simulink model "Mod5Counter"  (R2020a)
settings: Solver=VariableStepAuto  StartTime=0.0  StopTime=10.0  RelTol=1e-3
settings Model: Creator=Admin  LastModifiedBy=Admin

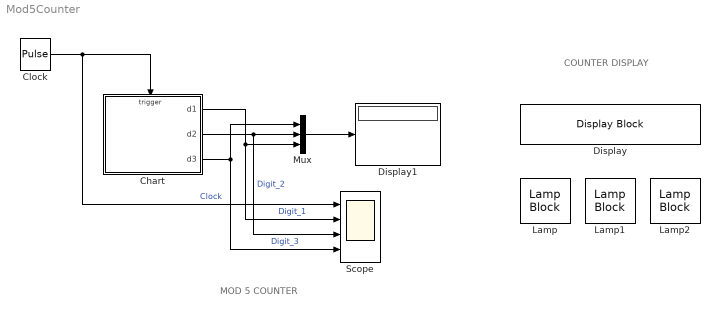
== system Mod5Counter ==
  note: MOD 5 COUNTER
  note: COUNTER DISPLAY
  Chart : Stateflow chart  TreatAsAtomicUnit=on
  Clock : DiscretePulseGenerator  PulseType=Time based  Period=0.5  PulseWidth=50
  Display : DisplayBlock  LabelPosition=Hide  Format=short  Transparency=1
  Display1 : Display
  Lamp : LampBlock
  Lamp1 : LampBlock
  Lamp2 : LampBlock
  Mux : Mux  Inputs=3
  Scope : Scope  NumInputPorts=4
  wires:
  Clock/1 -> Scope/1, Chart/Trigger  "Clock"
  Chart/1(d1) -> Mux/3, Scope/2  "Digit_1"
  Chart/2(d2) -> Mux/2, Scope/3  "Digit_2"
  Chart/3(d3) -> Mux/1, Scope/4  "Digit_3"
  Mux/1 -> Display1/1

== stateflow chart Mod5Counter/Chart ==
  state digit1 [parallel]
    settings: executionOrder=1
    state Zero
      en: d1 = 0;
    state One
      en: d1 = 1;
    state Two
      en: d1 = 2;
    (default) -> digit1.Zero
    digit1.Zero -> digit1.One : inc1
    digit1.One -> digit1.Zero [order 1] : [d2 == 1]/{inc3}
    Two -> digit1.Zero : inc1/{inc2}
    digit1.One -> Two [order 2] : inc1
  state digit2 [parallel]
    settings: executionOrder=2
    state Zero
      en: d2 = 0;
    state One
      en: d2 = 1;
    (default) -> digit2.Zero
    digit2.Zero -> digit2.One : inc2
    digit2.One -> digit2.Zero : inc3
  state digit3 [parallel]
    settings: executionOrder=3
    state Zero
      en: d3= 0;
    (default) -> digit3.Zero
  data: d1 output; d2 output; d3 output
  events: inc1 input RISING_EDGE_EVENT; inc2 local FUNCTION_CALL_EVENT; inc3 local FUNCTION_CALL_EVENT
